simulink model "simulationCapstone"  (R2022b)
settings: Solver=VariableStepAuto  StartTime=0.0  StopTime=10  RelTol=1e-3
values from neighbouring files (symbols this model uses):
  Bchopped = [C3 0 0 0; 0 C3 0 0]    [capstoneINIT.m]    (also in newPendulumControl.m; timevaryingSYS.m)
  C1 = CNa*leverArm*(0.5*density*v^2)/I    (= -484.328867428)    [capstoneINIT.m]    (also in controlMathtestScript.m = 14; newPendulumControl.m = 14.61; timevaryingSYS.m = CNa*leverArm*(0.5*density*v0^2)/I)
  C2 = -((CNa*(leverArm^2)*(0.5*density*v)/I)+(0.055*0.1*0.1))    (= -0.323435911619)    [capstoneINIT.m]    (also in controlMathtestScript.m = -0.121082216857; newPendulumControl.m = -0.121082216857; timevaryingSYS.m = -((CNa*(leverArm^2)*(0.5*density*v0)/I)-(0.055*0.1*0.1)))
undefined symbols (not defined in the file or in its folder): K1
libraries: slctrlblks x1, simulink x1
settings Model: Creator=rishi  LastModifiedBy=rishi

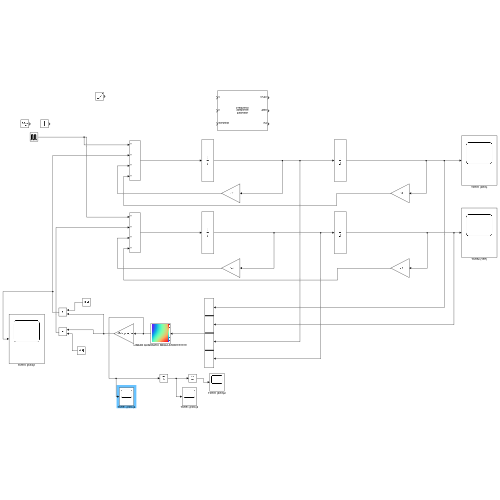
[thumbnail: Simulink's stored preview of the top-level diagram]
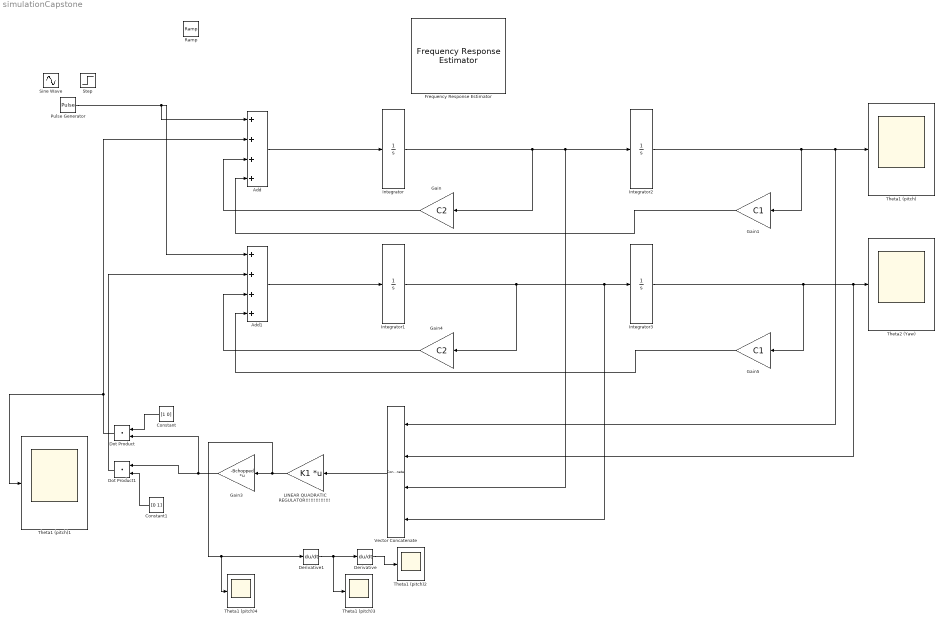
== system simulationCapstone ==
  Add : Sum  Inputs=++++
  Add1 : Sum  Inputs=++++
  Constant : Constant  Value=[1 0]
  Constant1 : Constant  Value=[0 1]
  Derivative : Derivative
  Derivative1 : Derivative
  Dot Product : DotProduct  OutDataTypeStr=Inherit: Inherit via internal rule
  Dot Product1 : DotProduct  OutDataTypeStr=Inherit: Inherit via internal rule
  Frequency Response Estimator : slctrlblks/Frequency Response Estimator  DiscreteTs=0.1  OutputMode=control action + perturbation  BlockDataType=double  SineSource=Block parameters  Frequencies=[0.5 1 2]  FreqUnits=rad/s  Amplitudes=1  NumOfFreq=3  ExperimentMode=Sinestream  NumOfSetPeriod=2  NumOfEstPeriod=4  NumOfSlowestPeriod=3  EstimationMode=Online  UseBodePlot=off  BaselinePlant=[]  PlotRefreshFactor=100  BodePlotChoice=VariantNull  ExperimentChoice=VariantSS  OutputChoice=VariantCandD
  Gain : Gain  Gain=C2
  Gain1 : Gain  Gain=C1
  Gain3 : Gain  Gain=-Bchopped  Multiplication=Matrix(K*u)
  Gain4 : Gain  Gain=C2
  Gain5 : Gain  Gain=C1
  Integrator{,1..3} (4 alike) : Integrator
  "LINEAR QUADRATIC REGULATOR!!!!!!!!!!!!!!! " : Gain  Gain=K1  Multiplication=Matrix(K*u)
      mask Display: image('/Users/rishi/Desktop/Screen Shot 2022-10-09 at 7.35.45 PM.png'); % Use "Edit Image" on toolstrip to change.
  Pulse Generator : DiscretePulseGenerator  PulseType=Time based  Amplitude=150  Period=10
  Ramp : simulink/Sources/Ramp  slope=1  start=0  InitialOutput=0
  Sine Wave : Sin  Amplitude=100  SampleTime=0
  Step : Step  After=500  SampleTime=0
  Theta1 (pitch){,1..4} (5 alike) : Scope
  Theta2 (Yaw) : Scope
  Vector Concatenate : Concatenate  NumInputs=4
  wires:
  Vector Concatenate/1 -> "LINEAR QUADRATIC REGULATOR!!!!!!!!!!!!!!! "/1
  Integrator/1 -> Gain/1, Vector Concatenate/3, Integrator2/1
  Add1/1 -> Integrator1/1
  Integrator1/1 -> Gain4/1, Vector Concatenate/4, Integrator3/1
  Add/1 -> Integrator/1
  Integrator3/1 -> Gain5/1, Vector Concatenate/2, Theta2 (Yaw)/1
  Integrator2/1 -> Gain1/1, Vector Concatenate/1, Theta1 (pitch)/1
  Gain1/1 -> Add/4
  Gain/1 -> Add/3
  Gain5/1 -> Add1/4
  Gain4/1 -> Add1/3
  Dot Product/1 -> Theta1 (pitch)1/1, Add/2
  Dot Product1/1 -> Add1/2
  "LINEAR QUADRATIC REGULATOR!!!!!!!!!!!!!!! "/1 -> Theta1 (pitch)4/1, Derivative1/1, Gain3/1
  Constant1/1 -> Dot Product1/2
  Constant/1 -> Dot Product/1
  Gain3/1 -> Dot Product/2, Dot Product1/1
  Pulse Generator/1 -> Add1/1, Add/1
  Derivative1/1 -> Theta1 (pitch)3/1, Derivative/1
  Derivative/1 -> Theta1 (pitch)2/1
